simulink model "PMSM_Control_model"  (R2023a)
settings: Solver=VariableStepAuto  StartTime=0.0  StopTime=1  RelTol=1e-3
values from neighbouring files (symbols this model uses):
  B = 0.00008    (= 8e-05)    [PMSM_set.m]
  J = 0.000028    (= 2.8e-05)    [PMSM_set.m]
  Kac = 1 / Kpc    (= 0.000361141206212)    [PMSM_set.m]
  Kas = 0    [PMSM_set.m]
  Kic = 2394    [PMSM_set.m]
  Kis = 700    [PMSM_set.m]
  Kpc = 2769    [PMSM_set.m]
  Kps = 10    [PMSM_set.m]
  Kt = (3/2) * np * Psi_f    (= 0.035560716)    [PMSM_set.m]
  pxyz = sqrt(3) * Tsw / Vdc    [PMSM_set.m]
  Rs = 0.89    [PMSM_set.m]
  Te_rated = P_rated / w_syn    (= 0.203718327158)    [PMSM_set.m]
  Tsw = 1 / fsw    (= 0.00237529691211)    [PMSM_set.m]
  V_max = sqrt(2) / sqrt(3) * V_rated    [PMSM_set.m]
  Vdc = 28    [PMSM_set.m]
libraries: simulink x4, slpidlib x3, spsDCVoltageSourceLib x1, mcbpmsmnonlinearlib x1, spsPermanentMagnetSynchronousMachineLib x1, spsSVPWMGenerator2LevelLib x1, spsUniversalBridgeLib x1, spsabctodq0Lib x1, spsdq0toabcLib x1, sps_lib x1
settings Model: Creator=涂钱龙  LastModifiedBy=涂钱龙

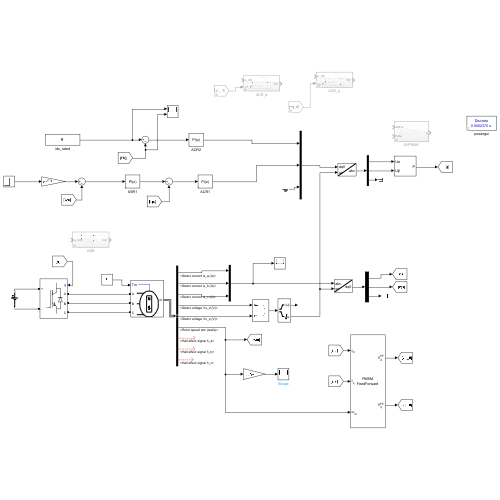
[thumbnail: Simulink's stored preview of the top-level diagram]
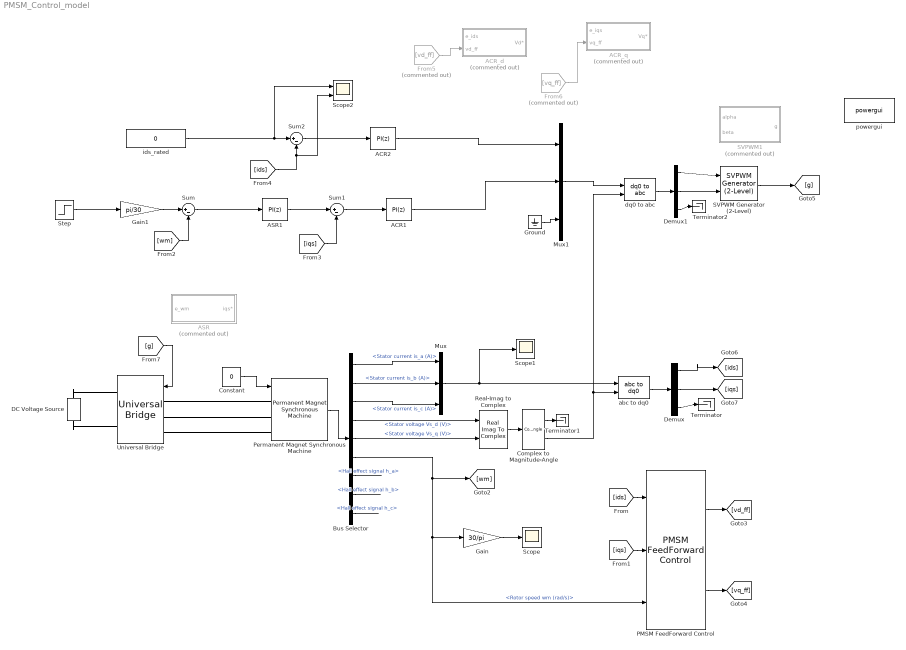
== system PMSM_Control_model ==
  ACR1 : slpidlib/PID Controller  Controller=PI  Form=Parallel  TimeDomain=Discrete-time  UseExternalTs=off  SampleTime=-1  IntegratorMethod=Forward Euler  FilterMethod=Forward Euler  ControllerParametersSource=internal  P=Kpc  I=Kic  UseKiTs=off  D=0  N=100  UseFilter=on  TunerSelectOption=Transfer Function Based (PID Tuner App)  InitialConditionSource=internal  InitialConditionForIntegrator=0  InitialConditionForFilter=0  DifferentiatorICPrevScaledInput=0  ExternalReset=none  TrackingMode=off  Kt=1  LimitOutput=off  SatLimitsSource=internal  UpperSaturationLimit=inf  LowerSaturationLimit=-inf  LinearizeAsGain=off  AntiWindupMode=none  Kb=1  LimitIntegrator=off  UpperIntegratorSaturationLimit=inf  LowerIntegratorSaturationLimit=-inf  POutMin=[]  POutMax=[]  IOutMin=[]  IOutMax=[]  DOutMin=[]  DOutMax=[]  NOutMin=[]  NOutMax=[]  SumOutMin=[]  SumOutMax=[]  SaturationOutMin=[]  SaturationOutMax=[]  PParamMin=[]  PParamMax=[]  IParamMin=[]  IParamMax=[]  DParamMin=[]  DParamMax=[]  NParamMin=[]  NParamMax=[]  KbParamMin=[]  KbParamMax=[]  KtParamMin=[]  KtParamMax=[]  KbOutMin=[]  KbOutMax=[]  KtOutMin=[]  KtOutMax=[]  IntegratorOutMin=[]  IntegratorOutMax=[]  FilterOutMin=[]  FilterOutMax=[]  SumI1OutMin=[]  SumI1OutMax=[]  SumI2OutMin=[]  SumI2OutMax=[]  SumI3OutMin=[]  SumI3OutMax=[]  SumI4OutMin=[]  SumI4OutMax=[]  SumDOutMin=[]  SumDOutMax=[]  DifferentiatorOutMin=[]  DifferentiatorOutMax=[]  FilterDiffOutCoefMin=[]  FilterDiffOutCoefMax=[]  ReciprocalOutMin=[]  ReciprocalOutMax=[]  SumDenOutMin=[]  SumDenOutMax=[]  SumNumOutMin=[]  SumNumOutMax=[]  DivideOutMin=[]  DivideOutMax=[]  UdiffTsProdOutMin=[]  UdiffTsProdOutMax=[]  NTsProdOutMin=[]  NTsProdOutMax=[]  UintegralTsProdOutMin=[]  UintegralTsProdOutMax=[]  UngainTsProdOutMin=[]  UngainTsProdOutMax=[]  ClampingZeroOutDataTypeStr=Inherit: Inherit via back propagation  ClampingZeroOutMin=[]  ClampingZeroOutMax=[]  FilterDenConstantOutDataTypeStr=Inherit: Inherit via back propagation  FilterDenConstantOutMin=[]  FilterDenConstantOutMax=[]  PCopyOutDataTypeStr=Inherit: Inherit via back propagation  PCopyOutMin=[]  PCopyOutMax=[]  NCopyOutDataTypeStr=Inherit: Inherit via back propagation  NCopyOutMin=[]  NCopyOutMax=[]  IntegratorContinuousStateAttributes=''  IntegratorStateMustResolveToSignalObject=off  IntegratorRTWStateStorageClass=Auto  FilterContinuousStateAttributes=''  FilterStateMustResolveToSignalObject=off  FilterRTWStateStorageClass=Auto  ParallelPVariant=InternalParameters  IdealPVariant=Disabled  IVariant=InternalParameters  DVariant=Disabled  IntegratorVariant=Discrete  SatVariant=Disabled  AWVariant=Passthrough  PCopyVariant=Disabled  TRVariant=Disabled  FdbkBlocksVariant=Forward  IdealPFdbkVariant=Disabled  SatFdbkVariant=Disabled  DerivativeFilterVariant=Disabled  NVariant=Disabled  NCopyVariant=Disabled_SignalSpec  FilterICVariant=Disabled  IntegratorICVariant=InternalICs  ExternalResetVariant=Disabled  TRSumVariant=Passthrough  SumFdbkVariant=Disabled  SumVariant=Sum_PI  TsampFilterVariant=InternalTs  TsampNgainVariant=Passthrough  TsampIntegralVariant=Disabled_SignalSpec  ExternalSaturationOutDataTypeStr=Inherit: Same as second input
      settings: LibrarySourceBlock=simulink/Discrete/Discrete PID Controller
  ACR2 : slpidlib/PID Controller  Controller=PI  Form=Parallel  TimeDomain=Discrete-time  UseExternalTs=off  SampleTime=-1  IntegratorMethod=Forward Euler  FilterMethod=Forward Euler  ControllerParametersSource=internal  P=Kpc  I=Kic  UseKiTs=off  D=0  N=100  UseFilter=on  TunerSelectOption=Transfer Function Based (PID Tuner App)  InitialConditionSource=internal  InitialConditionForIntegrator=0  InitialConditionForFilter=0  DifferentiatorICPrevScaledInput=0  ExternalReset=none  TrackingMode=off  Kt=1  LimitOutput=off  SatLimitsSource=internal  UpperSaturationLimit=inf  LowerSaturationLimit=-inf  LinearizeAsGain=off  AntiWindupMode=none  Kb=1  LimitIntegrator=off  UpperIntegratorSaturationLimit=inf  LowerIntegratorSaturationLimit=-inf  POutMin=[]  POutMax=[]  IOutMin=[]  IOutMax=[]  DOutMin=[]  DOutMax=[]  NOutMin=[]  NOutMax=[]  SumOutMin=[]  SumOutMax=[]  SaturationOutMin=[]  SaturationOutMax=[]  PParamMin=[]  PParamMax=[]  IParamMin=[]  IParamMax=[]  DParamMin=[]  DParamMax=[]  NParamMin=[]  NParamMax=[]  KbParamMin=[]  KbParamMax=[]  KtParamMin=[]  KtParamMax=[]  KbOutMin=[]  KbOutMax=[]  KtOutMin=[]  KtOutMax=[]  IntegratorOutMin=[]  IntegratorOutMax=[]  FilterOutMin=[]  FilterOutMax=[]  SumI1OutMin=[]  SumI1OutMax=[]  SumI2OutMin=[]  SumI2OutMax=[]  SumI3OutMin=[]  SumI3OutMax=[]  SumI4OutMin=[]  SumI4OutMax=[]  SumDOutMin=[]  SumDOutMax=[]  DifferentiatorOutMin=[]  DifferentiatorOutMax=[]  FilterDiffOutCoefMin=[]  FilterDiffOutCoefMax=[]  ReciprocalOutMin=[]  ReciprocalOutMax=[]  SumDenOutMin=[]  SumDenOutMax=[]  SumNumOutMin=[]  SumNumOutMax=[]  DivideOutMin=[]  DivideOutMax=[]  UdiffTsProdOutMin=[]  UdiffTsProdOutMax=[]  NTsProdOutMin=[]  NTsProdOutMax=[]  UintegralTsProdOutMin=[]  UintegralTsProdOutMax=[]  UngainTsProdOutMin=[]  UngainTsProdOutMax=[]  ClampingZeroOutDataTypeStr=Inherit: Inherit via back propagation  ClampingZeroOutMin=[]  ClampingZeroOutMax=[]  FilterDenConstantOutDataTypeStr=Inherit: Inherit via back propagation  FilterDenConstantOutMin=[]  FilterDenConstantOutMax=[]  PCopyOutDataTypeStr=Inherit: Inherit via back propagation  PCopyOutMin=[]  PCopyOutMax=[]  NCopyOutDataTypeStr=Inherit: Inherit via back propagation  NCopyOutMin=[]  NCopyOutMax=[]  IntegratorContinuousStateAttributes=''  IntegratorStateMustResolveToSignalObject=off  IntegratorRTWStateStorageClass=Auto  FilterContinuousStateAttributes=''  FilterStateMustResolveToSignalObject=off  FilterRTWStateStorageClass=Auto  ParallelPVariant=InternalParameters  IdealPVariant=Disabled  IVariant=InternalParameters  DVariant=Disabled  IntegratorVariant=Discrete  SatVariant=Disabled  AWVariant=Passthrough  PCopyVariant=Disabled  TRVariant=Disabled  FdbkBlocksVariant=Forward  IdealPFdbkVariant=Disabled  SatFdbkVariant=Disabled  DerivativeFilterVariant=Disabled  NVariant=Disabled  NCopyVariant=Disabled_SignalSpec  FilterICVariant=Disabled  IntegratorICVariant=InternalICs  ExternalResetVariant=Disabled  TRSumVariant=Passthrough  SumFdbkVariant=Disabled  SumVariant=Sum_PI  TsampFilterVariant=InternalTs  TsampNgainVariant=Passthrough  TsampIntegralVariant=Disabled_SignalSpec  ExternalSaturationOutDataTypeStr=Inherit: Same as second input
      settings: LibrarySourceBlock=simulink/Discrete/Discrete PID Controller
  ACR_d : Subsystem  Commented=on
  ACR_q : Subsystem  Commented=on
  ASR : Subsystem  Commented=on
  ASR1 : slpidlib/PID Controller  Controller=PI  Form=Parallel  TimeDomain=Discrete-time  UseExternalTs=off  SampleTime=-1  IntegratorMethod=Forward Euler  FilterMethod=Forward Euler  ControllerParametersSource=internal  P=Kps  I=Kis  UseKiTs=off  D=0  N=100  UseFilter=on  TunerSelectOption=Transfer Function Based (PID Tuner App)  InitialConditionSource=internal  InitialConditionForIntegrator=0  InitialConditionForFilter=0  DifferentiatorICPrevScaledInput=0  ExternalReset=none  TrackingMode=off  Kt=1  LimitOutput=off  SatLimitsSource=internal  UpperSaturationLimit=inf  LowerSaturationLimit=-inf  LinearizeAsGain=off  AntiWindupMode=none  Kb=1  LimitIntegrator=off  UpperIntegratorSaturationLimit=inf  LowerIntegratorSaturationLimit=-inf  POutMin=[]  POutMax=[]  IOutMin=[]  IOutMax=[]  DOutMin=[]  DOutMax=[]  NOutMin=[]  NOutMax=[]  SumOutMin=[]  SumOutMax=[]  SaturationOutMin=[]  SaturationOutMax=[]  PParamMin=[]  PParamMax=[]  IParamMin=[]  IParamMax=[]  DParamMin=[]  DParamMax=[]  NParamMin=[]  NParamMax=[]  KbParamMin=[]  KbParamMax=[]  KtParamMin=[]  KtParamMax=[]  KbOutMin=[]  KbOutMax=[]  KtOutMin=[]  KtOutMax=[]  IntegratorOutMin=[]  IntegratorOutMax=[]  FilterOutMin=[]  FilterOutMax=[]  SumI1OutMin=[]  SumI1OutMax=[]  SumI2OutMin=[]  SumI2OutMax=[]  SumI3OutMin=[]  SumI3OutMax=[]  SumI4OutMin=[]  SumI4OutMax=[]  SumDOutMin=[]  SumDOutMax=[]  DifferentiatorOutMin=[]  DifferentiatorOutMax=[]  FilterDiffOutCoefMin=[]  FilterDiffOutCoefMax=[]  ReciprocalOutMin=[]  ReciprocalOutMax=[]  SumDenOutMin=[]  SumDenOutMax=[]  SumNumOutMin=[]  SumNumOutMax=[]  DivideOutMin=[]  DivideOutMax=[]  UdiffTsProdOutMin=[]  UdiffTsProdOutMax=[]  NTsProdOutMin=[]  NTsProdOutMax=[]  UintegralTsProdOutMin=[]  UintegralTsProdOutMax=[]  UngainTsProdOutMin=[]  UngainTsProdOutMax=[]  ClampingZeroOutDataTypeStr=Inherit: Inherit via back propagation  ClampingZeroOutMin=[]  ClampingZeroOutMax=[]  FilterDenConstantOutDataTypeStr=Inherit: Inherit via back propagation  FilterDenConstantOutMin=[]  FilterDenConstantOutMax=[]  PCopyOutDataTypeStr=Inherit: Inherit via back propagation  PCopyOutMin=[]  PCopyOutMax=[]  NCopyOutDataTypeStr=Inherit: Inherit via back propagation  NCopyOutMin=[]  NCopyOutMax=[]  IntegratorContinuousStateAttributes=''  IntegratorStateMustResolveToSignalObject=off  IntegratorRTWStateStorageClass=Auto  FilterContinuousStateAttributes=''  FilterStateMustResolveToSignalObject=off  FilterRTWStateStorageClass=Auto  ParallelPVariant=InternalParameters  IdealPVariant=Disabled  IVariant=InternalParameters  DVariant=Disabled  IntegratorVariant=Discrete  SatVariant=Disabled  AWVariant=Passthrough  PCopyVariant=Disabled  TRVariant=Disabled  FdbkBlocksVariant=Forward  IdealPFdbkVariant=Disabled  SatFdbkVariant=Disabled  DerivativeFilterVariant=Disabled  NVariant=Disabled  NCopyVariant=Disabled_SignalSpec  FilterICVariant=Disabled  IntegratorICVariant=InternalICs  ExternalResetVariant=Disabled  TRSumVariant=Passthrough  SumFdbkVariant=Disabled  SumVariant=Sum_PI  TsampFilterVariant=InternalTs  TsampNgainVariant=Passthrough  TsampIntegralVariant=Disabled_SignalSpec  ExternalSaturationOutDataTypeStr=Inherit: Same as second input
      settings: LibrarySourceBlock=simulink/Discrete/Discrete PID Controller
  Bus Selector : BusSelector  OutputSignals=Stator current is_a (A),Stator current is_b (A),Stator current is_c (A),Stator voltage Vs_d (V),Stator voltage Vs_q (V),Rotor speed wm (rad/s),Hall effect signal h_a,Hall effect signal h_b,Hall effect signal h_c
  Complex to Magnitude-Angle : ComplexToMagnitudeAngle
  Constant : Constant  Value=0
  DC Voltage Source : spsDCVoltageSourceLib/DC Voltage Source  Amplitude=Vdc  Measurements=None
  Demux : Demux  Outputs=3
  Demux1 : Demux  Outputs=3
  From5 : From  Commented=on  GotoTag=vd_ff
  From6 : From  Commented=on  GotoTag=vq_ff
  Gain : Gain  Gain=30/pi
  Gain1 : Gain  Gain=pi/30
  Ground : Ground
  Mux : Mux  Inputs=3
  Mux1 : Mux  Inputs=3
  PMSM FeedForward Control : mcbpmsmnonlinearlib/PMSM FeedForward Control  polePairs=4  nonLinearityChoice=Linear model with lumped parameters  Ld=0.2e-3  Lq=0.2e-3  FluxPM=6.4e-3  idVec=[-40, -20, 0, 20]  iqVec=[-40, -20, 0, 20, 40]  LdTable=0.2e-3 * ones(4, 5)  LqTable=0.2e-3 * ones(4, 5)  FluxPMTable=6.4e-3 * ones(4, 5)  FluxDTable=[-1.6,-1.6,-1.6,-1.6,-1.6;2.4,2.4,2.4,2.4,2.4;6.4,6.4,6.4,6.4,6.4;10.4,10.4,10.4,10.4,10.4]*1e-3  FluxQTable=[-8,-4,0,4,8;-8,-4,0,4,8;-8,-4,0,4,8;-8,-4,0,4,8]*1e-3  Vsat_input_select=Specify via dialog  v_sat=24/sqrt(3)  Units=Per-Unit (PU)  V_base=24/sqrt(3)  I_base=19.3  N_base=4107  scaledTables=on
      settings: LibrarySourceBlock=mcblib/Controls/Control Reference/PMSM FeedForward Control
  Permanent Magnet Synchronous Machine : spsPermanentMagnetSynchronousMachineLib/Permanent Magnet Synchronous Machine  NbPhases=3  FluxDistribution=Sinusoidal  RotorType=Round  MechanicalLoad=Torque Tm  PresetModel=No  ShowDetailedParameters=on  MeasurementBus=off  Resistance=Rs  Inductance=8.5e-3  dqInductances=[8.5e-3,8.5e-3]  La=Ld  MachineConstant=Flux linkage established by magnets (V.s)  Flux=Psi_f  VoltageCst=4.3  TorqueCst=0.035561  Flat=120  Mechanical=[J B 4 0]  PolePairs=4  InitialConditions=[0,0, 0,0]  InitialConditions5ph=[0 0 0 0 0 0]  RefAngle=90 degrees behind phase A axis (modified Park)  IterativeDiscreteModel=Trapezoidal non iterative  TsBlock=-1  TsPowergui=0
  Real-Imag to Complex : RealImagToComplex
  SVPWM Generator (2-Level) : spsSVPWMGenerator2LevelLib/SVPWM Generator (2-Level)  InputType=alpha-beta components  SwitchingPattern=Pattern #1  Fc=fsw  ParUref=[0.8 -30 50]  Ts=Tsw/10
  SVPWM1 : Subsystem  Commented=on
  Scope : Scope
  Scope1 : Scope
  Scope2 : Scope  NumInputPorts=2
  Step : Step  Time=0.4  Before=500  After=1400  SampleTime=0
  Sum : Sum  Inputs=|+-
  Sum1 : Sum  Inputs=|+-
  Sum2 : Sum  Inputs=|+-
  Terminator : Terminator
  Terminator1 : Terminator
  Terminator2 : Terminator
  Universal Bridge : spsUniversalBridgeLib/Universal Bridge  Arms=3  SnubberResistance=1e5  SnubberCapacitance=inf  Device=IGBT / Diodes  Ron=1e-3  Lon=0  ForwardVoltages="[  0  0  ]"  ForwardVoltage=0  GTOparameters=[ 10e-6 , 20e-6 ]  IGBTparameters=[ 1e-6 , 2e-6 ]  Measurements=None  Measurements_2=None  converterType=Rectifier
  abc to dq0 : spsabctodq0Lib/abc to dq0  Alignment=90 degrees behind phase A axis
  dq0 to abc : spsdq0toabcLib/dq0 to abc  Alignment=90 degrees behind phase A axis
  ids_rated : Constant  Value=0
  powergui : sps_lib/powergui  Priority=1  SimulationMode=Discrete  SampleTime=Tsw/10  frequency=60  Iterations=50  frequencyindice=0  Pbase=100e6  ErrMax=1e-4  UnitsV=kV  UnitsW=MW  buscounter=0  FunctionMessages=off  echomessages=off  EnableUseOfTLC=off  CurrentSourceSwitches=off  DisableSnubberDevices=off  DisableRonSwitches=off  DisableVfSwitches=off  DisplayEquations=off  AutomaticDiscreteSolvers=off  SolverType=Tustin/Backward Euler (TBE)  Interpol=off  ExternalGateDelay=off  methode=off  Ts=100  x0status=blocks  SPID=on  SwTol=0  HookPort=off  NonlinearTolerance=1e-4  nMaxIteration=100  ContinueOnMaxIteration=off  RestoreLinks=warning  ResistiveCurrentMeasurement=off  Frange=[0:2:500]  Ylog=off  Xlog=on  ShowGrid=off  save=off  variable=ZData  structure=0  ZoomFFT=off  StartTime=0.0  cycles=1  DisplayStyle=1  fundamental=60  FreqAxis=off  MaxFrequency=1000  frequencyindicesteady=1  RmsSteady=1  display=off
  wires:
  Permanent Magnet Synchronous Machine/1 -> Bus Selector/1
  Bus Selector/1 -> Mux/1  "<Stator current is_a (A)>"
  Bus Selector/2 -> Mux/2  "<Stator current is_b (A)>"
  Bus Selector/3 -> Mux/3  "<Stator current is_c (A)>"
  Mux/1 -> Scope1/1, abc to dq0/1
  [ids] -> PMSM FeedForward Control/1
  [iqs] -> PMSM FeedForward Control/2
  Bus Selector/6 -> [wm], Gain/1, PMSM FeedForward Control/3  "<Rotor speed wm (rad/s)>"
  Bus Selector/5 -> Real-Imag to Complex/2  "<Stator voltage Vs_q (V)>"
  Bus Selector/4 -> Real-Imag to Complex/1  "<Stator voltage Vs_d (V)>"
  Real-Imag to Complex/1 -> Complex to Magnitude-Angle/1
  Complex to Magnitude-Angle/1 -> Terminator1/1
  Complex to Magnitude-Angle/2 -> dq0 to abc/2, abc to dq0/2
  Gain/1 -> Scope/1
  From5/1 -> ACR_d/2(vd_ff)
  From6/1 -> ACR_q/2(vq_ff)
  [ids] -> Sum2/2, Scope2/2
  ids_rated/1 -> Sum2/1, Scope2/1
  [iqs] -> Sum1/2
  [wm] -> Sum/2
  Gain1/1 -> Sum/1
  Step/1 -> Gain1/1
  PMSM FeedForward Control/1 -> [vd_ff]
  PMSM FeedForward Control/2 -> [vq_ff]
  Ground/1 -> Mux1/3
  Mux1/1 -> dq0 to abc/1
  dq0 to abc/1 -> Demux1/1
  Demux1/1 -> SVPWM Generator (2-Level)/1
  Demux1/3 -> Terminator2/1
  Demux1/2 -> SVPWM Generator (2-Level)/2
  SVPWM Generator (2-Level)/1 -> [g]
  [g] -> Universal Bridge/1
  Constant/1 -> Permanent Magnet Synchronous Machine/1
  Sum/1 -> ASR1/1
  ASR1/1 -> Sum1/1
  Sum2/1 -> ACR2/1
  ACR2/1 -> Mux1/1
  Sum1/1 -> ACR1/1
  ACR1/1 -> Mux1/2
  abc to dq0/1 -> Demux/1
  Demux/1 -> [ids]
  Demux/2 -> [iqs]
  Demux/3 -> Terminator/1
  Bus Selector/7 -> ?  "<Hall effect signal h_a>"
  Bus Selector/8 -> ?  "<Hall effect signal h_b>"
  Bus Selector/9 -> ?  "<Hall effect signal h_c>"
  connections:
  Universal Bridge/LConn3 -- Permanent Magnet Synchronous Machine/LConn3
  Universal Bridge/LConn2 -- Permanent Magnet Synchronous Machine/LConn2
  Universal Bridge/LConn1 -- Permanent Magnet Synchronous Machine/LConn1
  DC Voltage Source/RConn1 -- Universal Bridge/RConn1
  DC Voltage Source/LConn1 -- Universal Bridge/RConn2

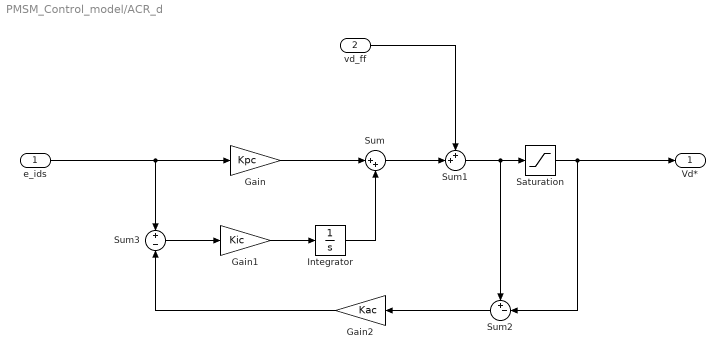
== system PMSM_Control_model/ACR_d ==
  e_ids : Inport
  vd_ff : Inport  Port=2
  Gain : Gain  Gain=Kpc
  Gain1 : Gain  Gain=Kic
  Gain2 : Gain  Gain=Kac
  Integrator : Integrator
  Saturation : Saturate  UpperLimit=V_max * 2  LowerLimit=-V_max * 2
  Sum : Sum  Inputs=|++
  Sum1 : Sum  Inputs=++|
  Sum2 : Sum  Inputs=+-|
  Sum3 : Sum  Inputs=+|-
  Vd* : Outport
  wires:
  Gain2/1 -> Sum3/2
  Sum3/1 -> Gain1/1
  Sum2/1 -> Gain2/1
  Saturation/1 -> Vd*/1, Sum2/2
  Sum1/1 -> Sum2/1, Saturation/1
  vd_ff/1 -> Sum1/1
  Sum/1 -> Sum1/2
  Integrator/1 -> Sum/2
  Gain/1 -> Sum/1
  Gain1/1 -> Integrator/1
  e_ids/1 -> Gain/1, Sum3/1

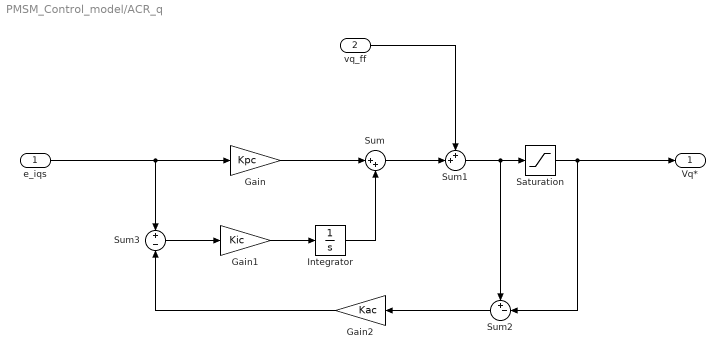
== system PMSM_Control_model/ACR_q ==
  e_iqs : Inport
  vq_ff : Inport  Port=2
  Gain : Gain  Gain=Kpc
  Gain1 : Gain  Gain=Kic
  Gain2 : Gain  Gain=Kac
  Integrator : Integrator
  Saturation : Saturate  UpperLimit=V_max * 2  LowerLimit=-V_max * 2
  Sum : Sum  Inputs=|++
  Sum1 : Sum  Inputs=++|
  Sum2 : Sum  Inputs=+-|
  Sum3 : Sum  Inputs=+|-
  Vq* : Outport
  wires:
  Gain2/1 -> Sum3/2
  Sum3/1 -> Gain1/1
  Sum2/1 -> Gain2/1
  Saturation/1 -> Vq*/1, Sum2/2
  Sum1/1 -> Sum2/1, Saturation/1
  vq_ff/1 -> Sum1/1
  Sum/1 -> Sum1/2
  Integrator/1 -> Sum/2
  Gain/1 -> Sum/1
  Gain1/1 -> Integrator/1
  e_iqs/1 -> Gain/1, Sum3/1

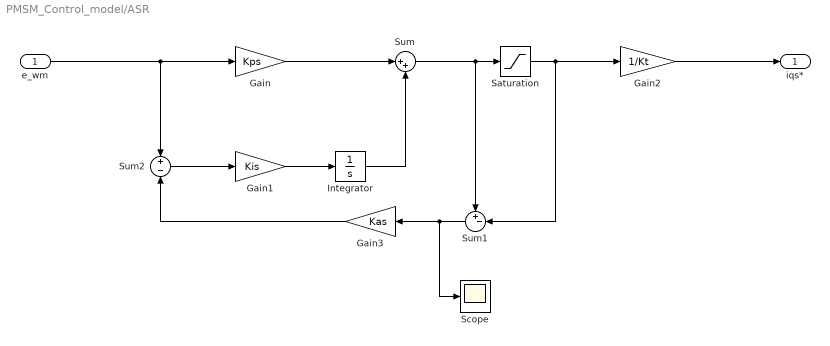
== system PMSM_Control_model/ASR ==
  e_wm : Inport
  Gain : Gain  Gain=Kps
  Gain1 : Gain  Gain=Kis
  Gain2 : Gain  Gain=1/Kt
  Gain3 : Gain  Gain=Kas
  Integrator : Integrator
  Saturation : Saturate  UpperLimit=Te_rated  LowerLimit=-Te_rated
  Scope : Scope
  Sum : Sum  Inputs=|++
  Sum1 : Sum  Inputs=+-|
  Sum2 : Sum  Inputs=+|-
  iqs* : Outport
  wires:
  Gain3/1 -> Sum2/2
  Sum2/1 -> Gain1/1
  Sum1/1 -> Scope/1, Gain3/1
  Gain2/1 -> iqs*/1
  Saturation/1 -> Gain2/1, Sum1/2
  Sum/1 -> Saturation/1, Sum1/1
  Integrator/1 -> Sum/2
  Gain/1 -> Sum/1
  Gain1/1 -> Integrator/1
  e_wm/1 -> Gain/1, Sum2/1

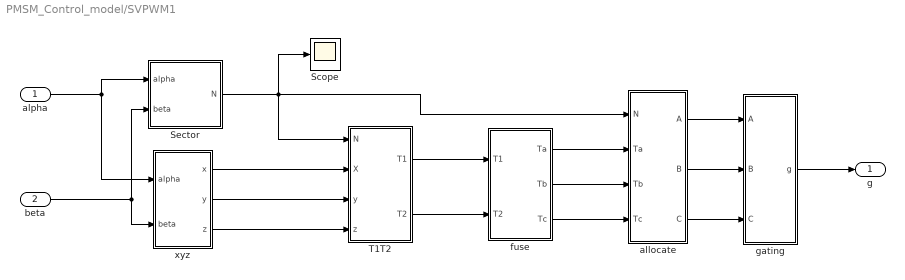
== system PMSM_Control_model/SVPWM1 ==
  alpha : Inport
  beta : Inport  Port=2
  Scope : Scope
  Sector : Subsystem
  T1T2 : Subsystem
  allocate : Subsystem
  fuse : Subsystem
  gating : Subsystem
  xyz : Subsystem
  g : Outport
  wires:
  gating/1(g) -> g/1
  beta/1 -> xyz/2(beta), Sector/2(beta)
  alpha/1 -> xyz/1(alpha), Sector/1(alpha)
  xyz/1(x) -> T1T2/2(X)
  fuse/1(Ta) -> allocate/2(Ta)
  Sector/1(N) -> allocate/1(N), Scope/1, T1T2/1(N)
  fuse/3(Tc) -> allocate/4(Tc)
  T1T2/2(T2) -> fuse/2(T2)
  xyz/3(z) -> T1T2/4(z)
  T1T2/1(T1) -> fuse/1(T1)
  xyz/2(y) -> T1T2/3(y)
  allocate/2(B) -> gating/2(B)
  allocate/1(A) -> gating/1(A)
  fuse/2(Tb) -> allocate/3(Tb)
  allocate/3(C) -> gating/3(C)

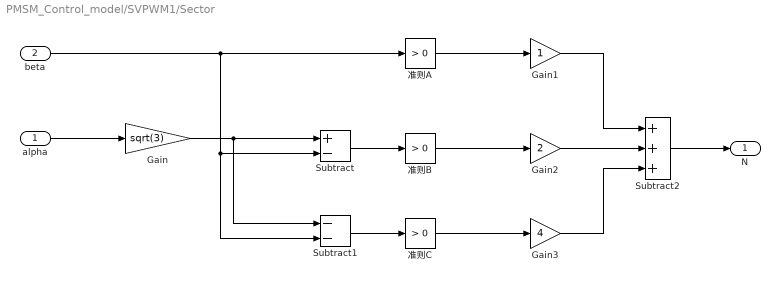
== system PMSM_Control_model/SVPWM1/Sector ==
  alpha : Inport
  beta : Inport  Port=2
  Gain : Gain  Gain=sqrt(3)
  Gain1 : Gain
  Gain2 : Gain  Gain=2
  Gain3 : Gain  Gain=4
  Subtract : Sum  Inputs=+-
  Subtract1 : Sum  Inputs=--
  Subtract2 : Sum  Inputs=+++
  准则A : simulink/Logic and Bit Operations/Compare To Constant  relop=>  const=0  OutDataTypeStr=boolean
  准则B : simulink/Logic and Bit Operations/Compare To Constant  relop=>  const=0  OutDataTypeStr=boolean
  准则C : simulink/Logic and Bit Operations/Compare To Constant  relop=>  const=0  OutDataTypeStr=boolean
  N : Outport
  wires:
  Subtract2/1 -> N/1
  Gain3/1 -> Subtract2/3
  Gain2/1 -> Subtract2/2
  Gain1/1 -> Subtract2/1
  准则A/1 -> Gain1/1
  准则B/1 -> Gain2/1
  准则C/1 -> Gain3/1
  Subtract1/1 -> 准则C/1
  Subtract/1 -> 准则B/1
  Gain/1 -> Subtract/1, Subtract1/1
  alpha/1 -> Gain/1
  beta/1 -> 准则A/1, Subtract/2, Subtract1/2

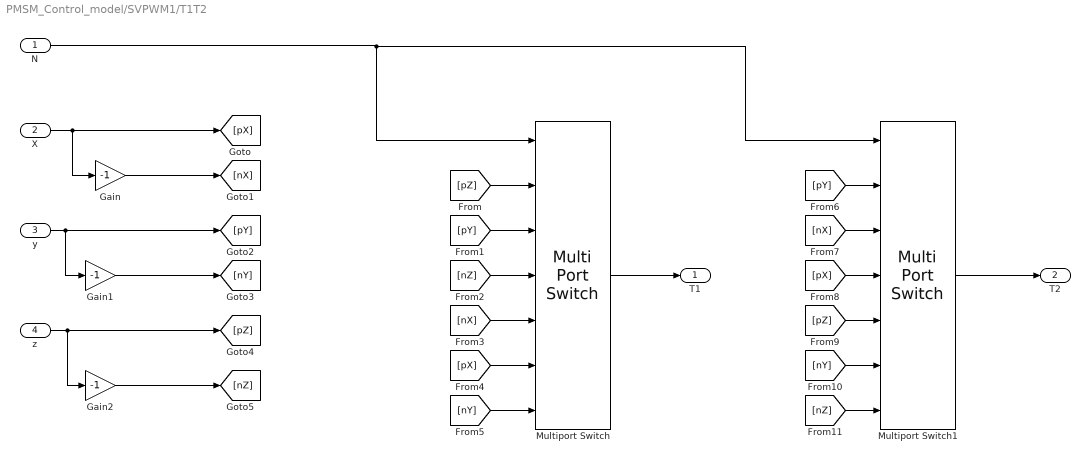
== system PMSM_Control_model/SVPWM1/T1T2 ==
  N : Inport
  X : Inport  Port=2
  y : Inport  Port=3
  z : Inport  Port=4
  Gain : Gain  Gain=-1
  Gain1 : Gain  Gain=-1
  Gain2 : Gain  Gain=-1
  Multiport Switch : MultiPortSwitch  Inputs=6  SaturateOnIntegerOverflow=off  InputSameDT=off
  Multiport Switch1 : MultiPortSwitch  Inputs=6  SaturateOnIntegerOverflow=off  InputSameDT=off
  T1 : Outport
  T2 : Outport  Port=2
  wires:
  [nZ] -> Multiport Switch1/7
  [nY] -> Multiport Switch1/6
  [pZ] -> Multiport Switch1/5
  [pX] -> Multiport Switch1/4
  [nX] -> Multiport Switch1/3
  [pY] -> Multiport Switch1/2
  [nY] -> Multiport Switch/7
  [pX] -> Multiport Switch/6
  [nX] -> Multiport Switch/5
  [nZ] -> Multiport Switch/4
  [pY] -> Multiport Switch/3
  [pZ] -> Multiport Switch/2
  N/1 -> Multiport Switch/1, Multiport Switch1/1
  Multiport Switch1/1 -> T2/1
  Multiport Switch/1 -> T1/1
  Gain2/1 -> [nZ]
  Gain1/1 -> [nY]
  Gain/1 -> [nX]
  z/1 -> [pZ], Gain2/1
  y/1 -> Gain1/1, [pY]
  X/1 -> Gain/1, [pX]

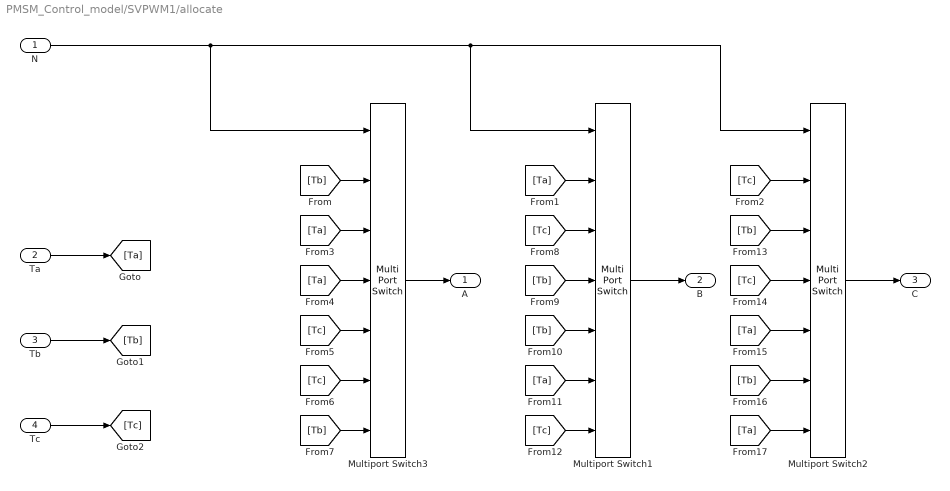
== system PMSM_Control_model/SVPWM1/allocate ==
  N : Inport
  Ta : Inport  Port=2
  Tb : Inport  Port=3
  Tc : Inport  Port=4
  Multiport Switch1 : MultiPortSwitch  Inputs=6  SaturateOnIntegerOverflow=off  InputSameDT=off
  Multiport Switch2 : MultiPortSwitch  Inputs=6  SaturateOnIntegerOverflow=off  InputSameDT=off
  Multiport Switch3 : MultiPortSwitch  Inputs=6  SaturateOnIntegerOverflow=off  InputSameDT=off
  A : Outport
  B : Outport  Port=2
  C : Outport  Port=3
  wires:
  [Ta] -> Multiport Switch2/7
  [Tb] -> Multiport Switch2/6
  [Ta] -> Multiport Switch2/5
  [Tc] -> Multiport Switch2/4
  [Tb] -> Multiport Switch2/3
  [Tc] -> Multiport Switch1/7
  [Ta] -> Multiport Switch1/6
  [Tb] -> Multiport Switch1/5
  [Tb] -> Multiport Switch1/4
  [Tc] -> Multiport Switch1/3
  [Tb] -> Multiport Switch3/7
  [Tc] -> Multiport Switch3/6
  [Tc] -> Multiport Switch3/5
  [Ta] -> Multiport Switch3/4
  [Ta] -> Multiport Switch3/3
  [Tc] -> Multiport Switch2/2
  [Ta] -> Multiport Switch1/2
  [Tb] -> Multiport Switch3/2
  N/1 -> Multiport Switch2/1, Multiport Switch1/1, Multiport Switch3/1
  Multiport Switch1/1 -> B/1
  Multiport Switch3/1 -> A/1
  Multiport Switch2/1 -> C/1
  Ta/1 -> [Ta]
  Tb/1 -> [Tb]
  Tc/1 -> [Tc]

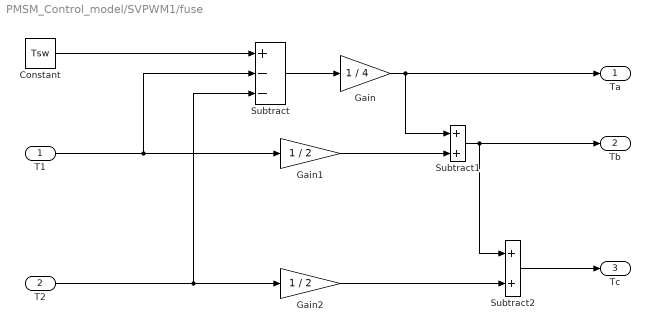
== system PMSM_Control_model/SVPWM1/fuse ==
  T1 : Inport
  T2 : Inport  Port=2
  Constant : Constant  Value=Tsw
  Gain : Gain  Gain=1 / 4
  Gain1 : Gain  Gain=1 / 2
  Gain2 : Gain  Gain=1 / 2
  Subtract : Sum  Inputs=+--
  Subtract1 : Sum
  Subtract2 : Sum
  Ta : Outport
  Tb : Outport  Port=2
  Tc : Outport  Port=3
  wires:
  Gain2/1 -> Subtract2/2
  Subtract2/1 -> Tc/1
  Subtract1/1 -> Tb/1, Subtract2/1
  Gain1/1 -> Subtract1/2
  Gain/1 -> Ta/1, Subtract1/1
  Subtract/1 -> Gain/1
  T2/1 -> Subtract/3, Gain2/1
  T1/1 -> Subtract/2, Gain1/1
  Constant/1 -> Subtract/1

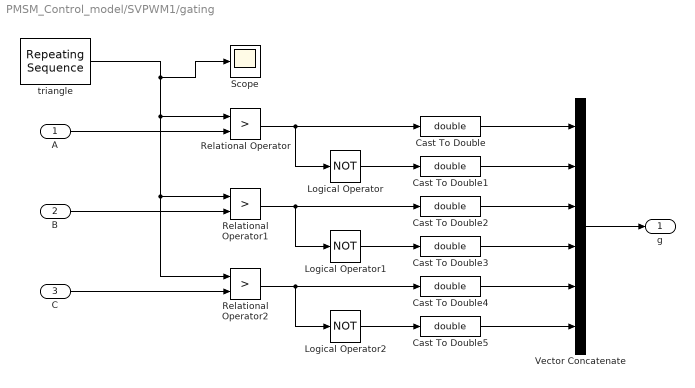
== system PMSM_Control_model/SVPWM1/gating ==
  A : Inport
  B : Inport  Port=2
  C : Inport  Port=3
  Cast To Double{,1..5} (6 alike) : DataTypeConversion  OutDataTypeStr=double  SaturateOnIntegerOverflow=off  RndMeth=Floor
  Logical Operator : Logic  Operator=NOT  AllPortsSameDT=off  OutDataTypeStr=boolean
  Logical Operator1 : Logic  Operator=NOT  AllPortsSameDT=off  OutDataTypeStr=boolean
  Logical Operator2 : Logic  Operator=NOT  AllPortsSameDT=off  OutDataTypeStr=boolean
  Relational Operator : RelationalOperator  Operator=>  OutDataTypeStr=boolean  RndMeth=Simplest  InputSameDT=off
  Relational Operator1 : RelationalOperator  Operator=>  OutDataTypeStr=boolean  RndMeth=Simplest  InputSameDT=off
  Relational Operator2 : RelationalOperator  Operator=>  OutDataTypeStr=boolean  RndMeth=Simplest  InputSameDT=off
  Scope : Scope
  Vector Concatenate : Concatenate  NumInputs=6
  triangle : simulink/Sources/Repeating Sequence  rep_seq_t=[0 Tsw/2 Tsw]  rep_seq_y=[0 Tsw/2 0]
  g : Outport
  wires:
  Vector Concatenate/1 -> g/1
  Cast To Double5/1 -> Vector Concatenate/6
  Cast To Double4/1 -> Vector Concatenate/5
  Cast To Double3/1 -> Vector Concatenate/4
  Cast To Double2/1 -> Vector Concatenate/3
  Cast To Double1/1 -> Vector Concatenate/2
  Cast To Double/1 -> Vector Concatenate/1
  Logical Operator2/1 -> Cast To Double5/1
  Logical Operator1/1 -> Cast To Double3/1
  Logical Operator/1 -> Cast To Double1/1
  Relational Operator2/1 -> Logical Operator2/1, Cast To Double4/1
  Relational Operator/1 -> Logical Operator/1, Cast To Double/1
  Relational Operator1/1 -> Logical Operator1/1, Cast To Double2/1
  C/1 -> Relational Operator2/2
  B/1 -> Relational Operator1/2
  A/1 -> Relational Operator/2
  triangle/1 -> Relational Operator1/1, Relational Operator2/1, Relational Operator/1, Scope/1

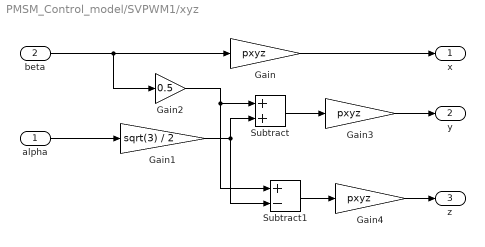
== system PMSM_Control_model/SVPWM1/xyz ==
  alpha : Inport
  beta : Inport  Port=2
  Gain : Gain  Gain=pxyz
  Gain1 : Gain  Gain=sqrt(3) / 2
  Gain2 : Gain  Gain=0.5
  Gain3 : Gain  Gain=pxyz
  Gain4 : Gain  Gain=pxyz
  Subtract : Sum
  Subtract1 : Sum  Inputs=+-
  x : Outport
  y : Outport  Port=2
  z : Outport  Port=3
  wires:
  Subtract1/1 -> Gain4/1
  Gain4/1 -> z/1
  Subtract/1 -> Gain3/1
  Gain3/1 -> y/1
  Gain1/1 -> Subtract1/2, Subtract/2
  Gain2/1 -> Subtract/1, Subtract1/1
  alpha/1 -> Gain1/1
  Gain/1 -> x/1
  beta/1 -> Gain/1, Gain2/1
